simulink model "position_controller"  (R2014b)
settings: Solver=FixedStepDiscrete  StartTime=0.0  StopTime=inf  FixedStep=sample_time  RelTol=1e-3
StartFcn:
  | tg.sampletime = correctedSampleTime;
settings Model: SimulationMode=external  BufferReuse=off  Creator=wmartin  LastModifiedBy=andrew
settings SolverCC: EnableConcurrentExecution=on
settings DataIOCC: LimitDataPoints=off  MaxDataPoints=1e7  SaveFormat=StructureWithTime  SignalLogging=off  DSMLogging=off
settings OptimizationCC: BlockReduction=off  OptimizeBlockIOStorage=off  BufferReuse=off  GlobalBufferReuse=off  ExpressionFolding=off  ExpressionDepthLimit=2147483647  LocalBlockOutputs=off  SimCompilerOptimization=On
settings DebuggingCC: UnderspecifiedInitializationDetection=Classic  MergeDetectMultiDrivingBlocksExec=none  StateNameClashWarn=warning
settings HardwareCC: ProdIntDivRoundTo=Zero  ProdEndianess=LittleEndian  ProdLongLongMode=on  ProdHWDeviceType=Generic->32-bit x86 compatible
settings ModelReferenceCC: UpdateModelReferenceTargets=IfOutOfDate  ModelReferenceNumInstancesAllowed=Single  ModelReferenceMinAlgLoopOccurrences=on
settings RTWCC: SystemTargetFile=slrt.tlc  TemplateMakefile=slrt_default_tmf  Description=Simulink Real-Time  RTWVerbose=off  ProcessScript=slrt_make_rtw_hook  RTWCompilerOptimization=On
settings CodeAppCC: MaxIdLength=256
settings TargetCC: CodeReplacementLibrary=XPC_BLAS  ParMdlRefBuildCompliant=on  ConcurrentExecutionCompliant=on  MatFileLogging=on  EnableShiftOperators=on  MATLABClassNameForMDSCustomization=xpcAperiodicCustomization

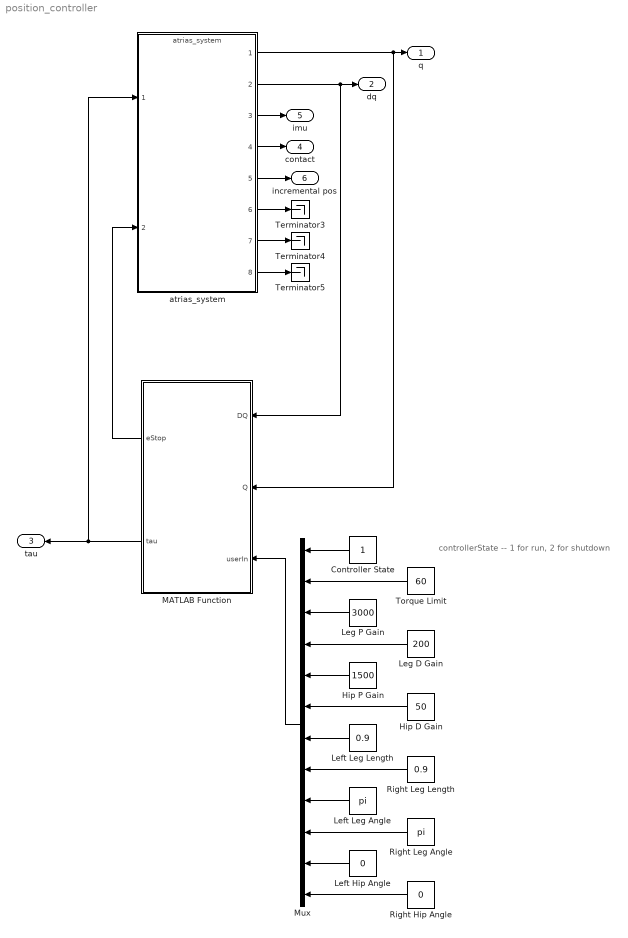
== system position_controller ==
  note: controllerState -- 1 for run, 2 for shutdown
  Controller State : Constant
  Hip D Gain : Constant  Value=50
  Hip P Gain : Constant  Value=1500
  Left Hip Angle : Constant  Value=0
  "Left Leg Angle " : Constant  Value=pi
  Left Leg Length : Constant  Value=0.9
  Leg D Gain : Constant  Value=200
  Leg P Gain : Constant  Value=3000
  MATLAB Function : MATLAB Function  TreatAsAtomicUnit=on
  Mux : Mux  Inputs=12
  Right Hip Angle : Constant  Value=0
  Right Leg Angle : Constant  Value=pi
  Right Leg Length : Constant  Value=0.9
  Terminator3 : Terminator
  Terminator4 : Terminator
  Terminator5 : Terminator
  Torque Limit : Constant  Value=60
  atrias_system : ModelReference  ModelNameDialog=atrias_system  SimulationMode=Normal  ModelReferenceVersion=1.2593  CopyOfModelName=atrias_system  DefaultDataLogging=on
  q : Outport
  dq : Outport  Port=2
  tau : Outport  Port=3
  contact : Outport  Port=4
  imu : Outport  Port=5
  incremental pos : Outport  Port=6
  wires:
  atrias_system/2 -> MATLAB Function/1(DQ), dq/1
  MATLAB Function/2(tau) -> atrias_system/1, tau/1
  atrias_system/3 -> imu/1
  atrias_system/1 -> MATLAB Function/2(Q), q/1
  atrias_system/4 -> contact/1
  atrias_system/5 -> incremental pos/1
  atrias_system/7 -> Terminator4/1
  atrias_system/6 -> Terminator3/1
  atrias_system/8 -> Terminator5/1
  MATLAB Function/1(eStop) -> atrias_system/2
  Mux/1 -> MATLAB Function/3(userIn)
  Controller State/1 -> Mux/1
  Torque Limit/1 -> Mux/2
  Leg P Gain/1 -> Mux/3
  Leg D Gain/1 -> Mux/4
  Hip P Gain/1 -> Mux/5
  Hip D Gain/1 -> Mux/6
  Left Leg Length/1 -> Mux/7
  Right Leg Length/1 -> Mux/8
  "Left Leg Angle "/1 -> Mux/9
  Right Leg Angle/1 -> Mux/10
  Left Hip Angle/1 -> Mux/11
  Right Hip Angle/1 -> Mux/12

== matlab function position_controller/MATLAB Function ==
  data: DQ input; eStop output; Q input; tau output; userIn input
function [eStop, tau] = positionController(DQ, Q, userIn)
%POSITIONCONTROLLER Control hip angles and leg angles and lengths
%
% Description:
%
% Notes:
% 	- State indexes (rBl rBm rAl rAm lBl lBm lAl lAm rHm lHm bR bY bP) 
%   - Input indexes (rB rA rH lB lA lH)
    
    % Constants for switch statements
    RUN = 1; SHUTDOWN = 2;
    
    % Initialize input vector to zeros
    u = zeros(6,1);
    
    % Set default emergency stop to false
    eStop = false;
    
    % Unpack inputs
    controllerState = userIn(1);
    tauLim = clamp(userIn(2), 0, 1000);
    kpl = clamp(userIn(3), 0, 10000);
    kdl = clamp(userIn(4), 0, 10000);
    kph = clamp(userIn(5), 0, 10000);
    kdh = clamp(userIn(6), 0, 10000);
    rLl = clamp(userIn(7), 0.5, 0.98);
    rRl = clamp(userIn(8), 0.5, 0.98);
    qLl = clamp(userIn(9), pi/2, 3*pi/2);
    qRl = clamp(userIn(10), pi/2, 3*pi/2);
    qLh = clamp(userIn(11), -0.2, 0.2);
    qRh = clamp(userIn(12), -0.2, 0.2);

	% Leg motor indices
    iqL = [2 4 6 8];
    iuL = [1 2 4 5];
    % Hip motor indices
    iqH = [9 10];
    iuH = [3 6];
    
    % Main controller state machine
    switch controllerState
        case RUN
            % Convert the desired leg length and leg angle to motor coordinates
            qRA = acos(rRl) - qRl;
            qRB = acos(rRl) + qRl;
            qLA = acos(rLl) - qLl;
            qLB = acos(rLl) + qLl;

            % Compute leg actuator torques using PD controller
            u(iuL) = ([qRB; qRA; qLB; qLA] - Q(iqL))*kpl + (0 - DQ(iqL))*kdl;

            % Compute hip actuator torques using PD controller
            u(iuH) = ([qRh; qLh] - Q(iqH))*kph + (0 - DQ(iqH))*kdh;

        case SHUTDOWN
            % Compute actuator torques using virtual damper
            u(iuL) = (0 - DQ(iqL))*kdl;
            u(iuH) = (0 - DQ(iqH))*kdh;

        otherwise; eStop = true;
    end % switch
    
    % Limit torques to be cautious
	tau = clamp(u, -tauLim, tauLim);
end % sampleController

function b = clamp(a, lim1, lim2)
%CLAMP Clamp value between two values.
	
	% Find which limit is min and max
	aMin = min(lim1, lim2);
	aMax = max(lim1, lim2);

	% Clamp value between limits
	b = max(min(a, aMax), aMin);
end % clamp
